simulink model "untitled"  (R2012b)
settings: Solver=ode45  StartTime=0.0  StopTime=2  RelTol=1e-3
undefined symbols (not defined in the file): A, B, C, D, sysd, Ts
settings Model: Creator=Juliano  LastModifiedBy=Juliano

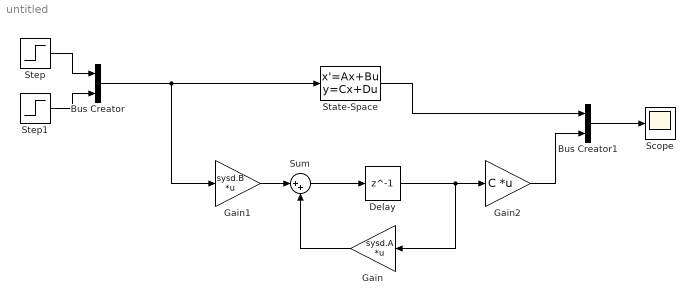
== system untitled ==
  Bus Creator : BusCreator  Inputs=2
  Bus Creator1 : BusCreator  Inputs=2
  Delay : Delay  DelayLength=1  SampleTime=Ts
  Gain : Gain  Gain=sysd.A  Multiplication=Matrix(K*u)
  Gain1 : Gain  Gain=sysd.B  Multiplication=Matrix(K*u)
  Gain2 : Gain  Gain=C  Multiplication=Matrix(K*u)
  Scope : Scope
  State-Space : StateSpace  A=A  B=B  C=C  D=D
  Step : Step  SampleTime=0
  Step1 : Step  SampleTime=0
  Sum : Sum  Inputs=|++
  wires:
  Step/1 -> Bus Creator/1
  Step1/1 -> Bus Creator/2
  Bus Creator/1 -> State-Space/1, Gain1/1
  State-Space/1 -> Bus Creator1/1
  Bus Creator1/1 -> Scope/1
  Gain1/1 -> Sum/1
  Gain/1 -> Sum/2
  Sum/1 -> Delay/1
  Delay/1 -> Gain2/1, Gain/1
  Gain2/1 -> Bus Creator1/2
